simulink model "SimulinkTCPA"  (R2020a)
settings: Solver=VariableStepAuto  StartTime=0.0  StopTime=100  RelTol=1e-3
settings Model: Creator=manth  LastModifiedBy=manth

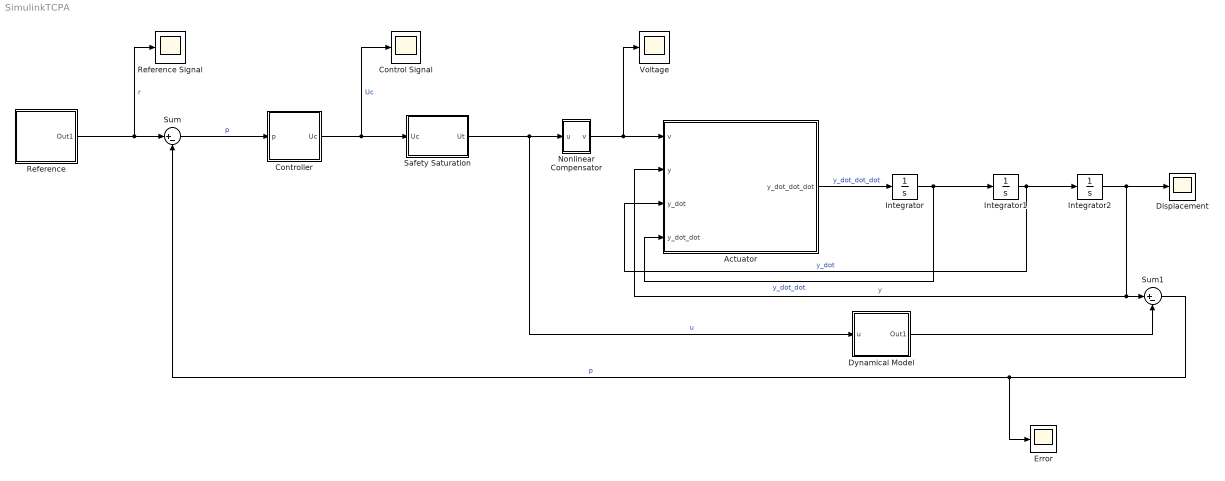
== system SimulinkTCPA ==
  Actuator : MATLAB Function  TreatAsAtomicUnit=on
  Control Signal : Scope
  Controller : Subsystem
  Displacement : Scope
  Dynamical Model : Subsystem
  Error : Scope
  Integrator : Integrator
  Integrator1 : Integrator
  Integrator2 : Integrator
  Nonlinear Compensator : Subsystem
  Reference : Subsystem
  Reference Signal : Scope
  Safety Saturation : MATLAB Function  TreatAsAtomicUnit=on
  Sum : Sum  Inputs=|+-
  Sum1 : Sum  Inputs=|+-
  Voltage : Scope
  wires:
  Safety Saturation/1(Ut) -> Dynamical Model/1(u), Nonlinear Compensator/1(u)  "u"
  Actuator/1(y_dot_dot_dot) -> Integrator/1  "y_dot_dot_dot"
  Integrator/1 -> Integrator1/1, Actuator/4(y_dot_dot)  "y_dot_dot"
  Integrator1/1 -> Actuator/3(y_dot), Integrator2/1  "y_dot"
  Integrator2/1 -> Displacement/1, Actuator/2(y), Sum1/1  "y"
  Sum1/1 -> Sum/2, Error/1  "p"
  Controller/1(Uc) -> Safety Saturation/1(Uc), Control Signal/1  "Uc"
  Sum/1 -> Controller/1(p)  "p"
  Dynamical Model/1(Out1) -> Sum1/2
  Nonlinear Compensator/1(v) -> Actuator/1(v), Voltage/1
  Reference/1(Out1) -> Reference Signal/1, Sum/1  "r"

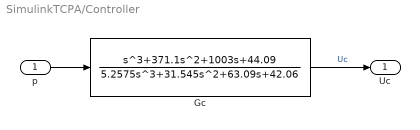
== system SimulinkTCPA/Controller ==
  p : Inport
  Gc : TransferFcn  Numerator=[1 371.1 1003 44.09]  Denominator=[5.2575 31.545 63.09 42.06]
  Uc : Outport
  wires:
  p/1 -> Gc/1
  Gc/1 -> Uc/1  "Uc"

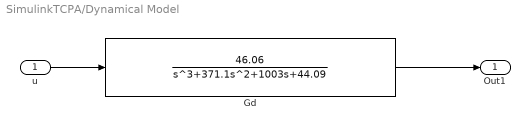
== system SimulinkTCPA/Dynamical Model ==
  u : Inport
  Gd : TransferFcn  Numerator=[46.06]  Denominator=[1 371.1 1003 44.09]
  Out1 : Outport
  wires:
  u/1 -> Gd/1
  Gd/1 -> Out1/1

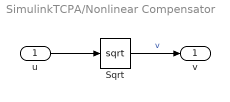
== system SimulinkTCPA/Nonlinear Compensator ==
  u : Inport
  Sqrt : Sqrt  SaturateOnIntegerOverflow=on
  v : Outport
  wires:
  u/1 -> Sqrt/1
  Sqrt/1 -> v/1  "v"

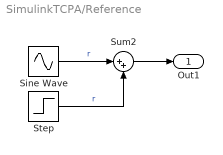
== system SimulinkTCPA/Reference ==
  Sine Wave : Sin  Amplitude=2  Frequency=0.62831853  SampleTime=0
  Step : Step  After=8  SampleTime=0
  Sum2 : Sum  Inputs=|++
  Out1 : Outport
  wires:
  Sine Wave/1 -> Sum2/1  "r"
  Step/1 -> Sum2/2  "r"
  Sum2/1 -> Out1/1

== matlab function SimulinkTCPA/Safety Saturation ==
  data: Uc input; Ut output
function Ut = Saturation(Uc)



if (100<Uc)
    Ut=100;
    
elseif (Uc<0)
    Ut=0;
else 
    Ut=Uc;
end

== matlab function SimulinkTCPA/Actuator ==
  data: v input; y input; y_dot_dot_dot output; y_dot input; y_dot_dot input
function y_dot_dot_dot = TCPA_Actuator(v,y,y_dot,y_dot_dot)

b0=42.09;
a0=44.09;
a1=1003;
a2=371.1;

y_dot_dot_dot = (b0*(v^2)) - (a2*y_dot_dot) - (a1*y_dot) - (a0*y);
